simulink model "commpassbandmod"  (R2021b)
settings: Solver=VariableStepDiscrete  StartTime=0.0  StopTime=0.02  RelTol=1e-3  EnableMultiTasking=on
InitFcn:
  | commpassbandmodParams.Fc = 2.5e6;
  | commpassbandmodParams.F1 = commpassbandmodParams.Fc/3+.5e5;
undefined symbols (not defined in the file or in its folder): comm, constellation
libraries: commutil2 x3, dspsrcs4 x3, commdigbbndpm3 x2, commfilt2 x2, commchan3 x1, commsink2 x1, commrandsrc3 x1
Description:
  | Passband Modulation
  | 
  | This model shows a straightforward way to perform passband modulation, by multiplying a modulated complex signal with a complex sine wave to perform frequency upconversion.
settings Model: Creator=The MathWorks, Inc.  LastModifiedBy=The MathWorks, Inc.
settings SolverCC: AlgebraicLoopSolver=TrustRegion  InsertRTBMode=Auto
settings DataIOCC: LimitDataPoints=on  SaveFormat=Array  SaveOutput=off  SignalLogging=off  SaveTime=off  ReturnWorkspaceOutputs=off
settings OptimizationCC: ExpressionDepthLimit=2147483647  InitFltsAndDblsToZero=on  EfficientMapNaN2IntZero=off  LifeSpan=inf
settings DebuggingCC: UnderspecifiedInitializationDetection=Classic  MergeDetectMultiDrivingBlocksExec=none  SolverPrmCheckMsg=warning  FcnCallInpInsideContextMsg=warning  AllowSymbolicDim=off  StateNameClashWarn=warning  SFUnexpectedBacktrackingDiag=warning  SFNoUnconditionalDefaultTransitionDiag=warning  SFExecutionAtInitializationDiag=none  SFMachineParentedDataDiag=warning  ArithmeticOperatorsInVariantConditions=warning
settings HardwareCC: ProdBitPerPointer=32  ProdBitPerSizeT=32  ProdBitPerPtrDiffT=32  ProdLargestAtomicFloat=None  ProdIntDivRoundTo=Undefined  ProdEndianess=Unspecified  ProdWordSize=32  ProdHWDeviceType=32-bit Generic
settings ModelReferenceCC: PropagateSignalLabelsOutOfModel=off
settings SFSimCC: SimUseLocalCustomCode=off  CustomCodeUndefinedFunction=UseInterfaceOnly
settings RTWCC: RTWUseLocalCustomCode=off
settings CodeAppCC: StateflowObjectComments=on
settings GRTTargetCC: TargetLangStandard=C89/C90 (ANSI)  CombineOutputUpdateFcns=off  GRTInterface=on
settings ConfigComp: CovMetricSettings=dw  CovSaveCumulativeToWorkspaceVar=on  CovSaveSingleToWorkspaceVar=on  CovExternalEMLEnable=off  CovSFcnEnable=off

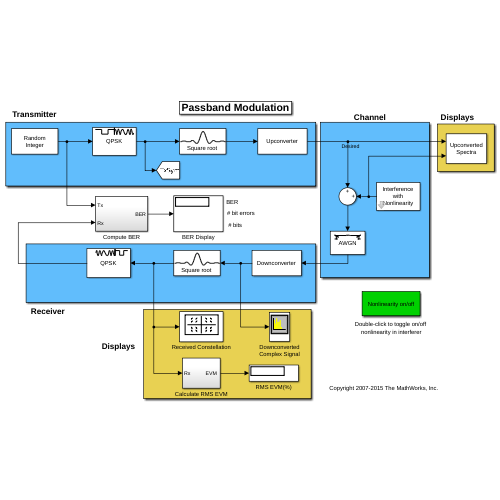
[thumbnail: Simulink's stored preview of the top-level diagram]
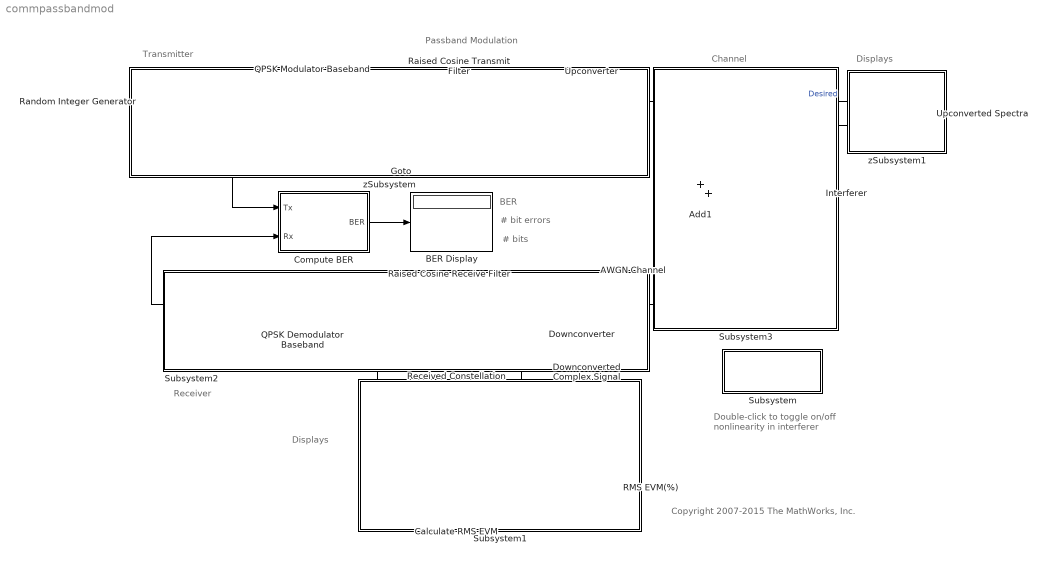
== system commpassbandmod ==
  note: Double-click to toggle on/off
      |  nonlinearity in interferer
  note: Passband Modulation
  note: Transmitter
  note: Receiver
  note: Channel
  note: Displays
  note: Displays
  note: BER
  note: # bit errors
  note: # bits
  note: Copyright 2007-2015 The MathWorks, Inc.
  AWGN Channel : commchan3/AWGN Channel  InputProcessing=Columns as channels (frame based)  seed=67  noiseMode="Signal to noise ratio  (Eb/No)"  EbNodB=8  EsNodB=10  SNRdB=10  bitsPerSym=2  Ps=1/(2*8)  Tsym=1e-6  variance=1
  Add1 : Sum  Inputs=|++
  BER Display : Display
  Calculate RMS EVM : Subsystem
  Compute BER : Subsystem
  Downconverted Complex Signal : SpectrumAnalyzer
  Downconverter : Subsystem
      mask Display: disp('Downconverter')
  Interferer : Subsystem  mask(Interference){nonlinOrder=3}
      mask prompts: nonlinOrder "Order of nonlinearity:"
      mask help: Generate out-of-band interference. Optionally process the interference with a third-order nonlinearity that creates an in-band harmonic.
      mask init:
      | if nonlinOrder == 1
      |     icontext = 'Interference\nwithout\nNonlinearity';
      | elseif nonlinOrder == 3
      |     icontext = 'Interference\nwith\nNonlinearity';
      | end
      mask Display: disp(icontext)
  QPSK Demodulator Baseband : commdigbbndpm3/QPSK Demodulator Baseband  OutType=Integer  DecType=Hard decision  VarSource=Dialog  Variance=1  Dec=Gray  Ph=pi/4  outDtype1=Inherit via internal rule  outDtype2=Inherit via internal rule  derotateFactorWordLen=16  derotateFactorDataTypeStr=Inherit: Same word length as input  derotateFactorLastDataTypeStr=Inherit: Same word length as input
  QPSK Modulator Baseband : commdigbbndpm3/QPSK Modulator Baseband  InType=Integer  Enc=Gray  Ph=pi/4  outDtype=double  outWordLen=16  outUDDataType=sfix(16)  outFracLenMode=Best precision  outFracLen=15  outDataTypeStr=double  outLastDataTypeStr=double
  RMS EVM(%) : Display
  Raised Cosine Receive Filter : commfilt2/Raised Cosine Receive Filter  filtType=Square root  R=0.2  filtSpan=8  N=8  downFactor=8  downOffset=0  filterGain=2  InputProcessing=Columns as channels (frame based)  RateOptions=Enforce single-rate processing  framing=Mute  checkCoeff=off  variableName=rcRxFilt1  currentFiltSpan=2*(4)  D=4  inputOffset=0  sampMode=Mute  saveAsFlag=0  rateMode=Downsampling  checkGain=User-specified  launchFVT=off  roundingMode=Floor  overflowMode=off  coeffDataTypeStr=Inherit: Same word length as input  coeffMin=[]  coeffMax=[]  coeffLastDataTypeStr=Inherit: Same word length as input  accumDataTypeStr=Inherit: Same as product output  accumLastDataTypeStr=Inherit: Same as product output  outputDataTypeStr=Inherit: Same as accumulator  outputMin=[]  outputMax=[]  outputLastDataTypeStr=Inherit: Same as accumulator
  Raised Cosine Transmit Filter : commfilt2/Raised Cosine Transmit Filter  filtType=Square root  R=0.2  filtSpan=8  N=8  filterGain=1  InputProcessing=Columns as channels (frame based)  RateOptions=Enforce single-rate processing  framing=Mute  checkCoeff=off  variableName=rcTxFilt1  checkGain=Normalized  sampMode=Mute  saveAsFlag=0  currentFiltSpan=2*(4)  D=4  launchFVT=off  roundingMode=Floor  overflowMode=off  coeffDataTypeStr=Inherit: Same word length as input  coeffMin=[]  coeffMax=[]  coeffLastDataTypeStr=Inherit: Same word length as input  outputDataTypeStr=Inherit: Same as accumulator  outputMin=[]  outputMax=[]  outputLastDataTypeStr=Inherit: Same as accumulator
  Random Integer Generator : commrandsrc3/Random Integer Generator  SetSize=4  SeedSource=Parameter  Seed=37  SampleTime=1e-6  SamplesPerFrame=100  OutputDataType=double  SimulateUsing=Interpreted execution
  Received Constellation : ConstellationDiagram  Tag=ScatterPlot
  Subsystem : Subsystem
      settings: OpenFcn=commpassbandmod_update
      mask Display: disp('Nonlinearity on/off')
  Subsystem1 : Subsystem
      mask Display: disp('')
  Subsystem2 : Subsystem
      mask Display: disp('')
  Subsystem3 : Subsystem
      mask Display: disp('')
  Upconverted Spectra : Subsystem
      mask Display: disp('Upconverted\nSpectra')
  Upconverter : Subsystem
      mask Display: disp('Upconverter')
  zSubsystem : Subsystem
      mask Display: disp('')
  zSubsystem1 : Subsystem
      mask Display: disp('')
  tag scope: TxSym=global
  wires:
  Random Integer Generator/1 -> QPSK Modulator Baseband/1, Compute BER/1(Tx)
  QPSK Modulator Baseband/1 -> Raised Cosine Transmit Filter/1, [TxSym]
  Compute BER/1(BER) -> BER Display/1
  QPSK Demodulator Baseband/1 -> Compute BER/2(Rx)
  AWGN Channel/1 -> Downconverter/1(In)
  Raised Cosine Transmit Filter/1 -> Upconverter/1(In)
  Raised Cosine Receive Filter/1 -> QPSK Demodulator Baseband/1, Calculate RMS EVM/1(Rx), Received Constellation/1
  Downconverter/1(Out) -> Raised Cosine Receive Filter/1, Downconverted Complex Signal/1
  Add1/1 -> AWGN Channel/1
  Calculate RMS EVM/1("EVM ") -> RMS EVM(%)/1
  Upconverter/1(Out) -> Add1/1, Upconverted Spectra/1(In1)  "Desired"
  Interferer/1(Out1) -> Add1/2, Upconverted Spectra/2(In2)

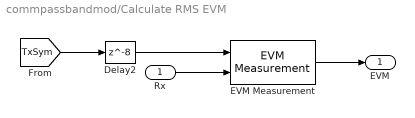
== system commpassbandmod/Calculate RMS EVM ==
  Rx : Inport
  Delay2 : Delay  DelayLength=8  InitialCondition=1  InputProcessing=Columns as channels (frame based)
  EVM Measurement : commutil2/EVM Measurement  Normalization=Average reference signal power  AverageConstellationPower=1  PeakConstellationPower=1  ReferenceSignalSource=Input port  ReferenceConstellation=constellation( comm.QPSKModulator )  MeasurementIntervalSource=Input length  MeasurementInterval=100  AveragingDimensions=1  MaximumEVMOutputPort=off  XPercentileEVMOutputPort=off  XPercentileValue=95  SymbolCountOutputPort=off  SimulateUsing=Interpreted execution
      settings: SourceProductBaseCode=CM
  "EVM " : Outport  VectorParamsAs1DForOutWhenUnconnected=off
  wires:
  Delay2/1 -> EVM Measurement/1
  [TxSym] -> Delay2/1
  Rx/1 -> EVM Measurement/2
  EVM Measurement/1 -> "EVM "/1

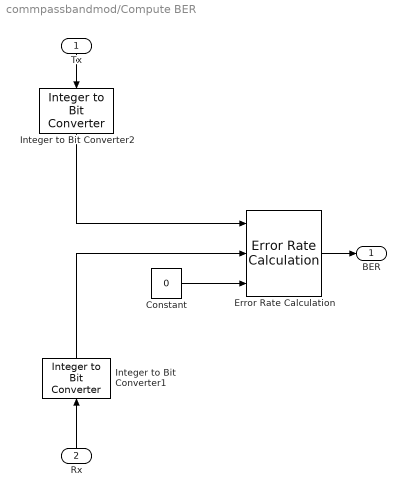
== system commpassbandmod/Compute BER ==
  Tx : Inport
  Rx : Inport  Port=2
  Constant : Constant  Value=0  SampleTime=1e-4
  Error Rate Calculation : commsink2/Error Rate Calculation  N=16  st_delay=0  cp_mode=Entire frame  subframe=[]  PMode=Port  WsName=ErrorVec  RsMode2=on  stop=off  numErr=100  maxBits=1e6
  Integer to Bit Converter1 : commutil2/Integer to Bit Converter  nbits=2  signedInputValues=Unsigned  bitOrder=MSB first  outDtype=boolean
  Integer to Bit Converter2 : commutil2/Integer to Bit Converter  nbits=2  signedInputValues=Unsigned  bitOrder=MSB first  outDtype=boolean
  BER : Outport  VectorParamsAs1DForOutWhenUnconnected=off
  wires:
  Integer to Bit Converter2/1 -> Error Rate Calculation/1
  Integer to Bit Converter1/1 -> Error Rate Calculation/2
  Tx/1 -> Integer to Bit Converter2/1
  Error Rate Calculation/1 -> BER/1
  Rx/1 -> Integer to Bit Converter1/1
  Constant/1 -> Error Rate Calculation/3

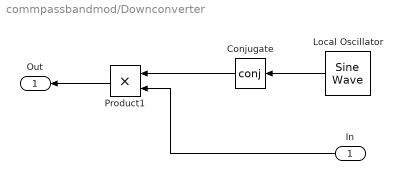
== system commpassbandmod/Downconverter ==
  In : Inport
  Conjugate : Math  Operator=conj  SignedPower=on  SaturateOnIntegerOverflow=on
  Local Oscillator : dspsrcs4/Sine Wave  Amplitude=1  Frequency=commpassbandmodParams.Fc  Phase=0  SampleMode=Discrete  OutComplex=Complex  CompMethod=Trigonometric fcn  TableSize=Speed  SampleTime=(1e-6) /8  SamplesPerFrame=800  ResetState=Restart at time zero  OutputFrames=off  dataType=double  wordLen=16  udDataType=sfix(16)  fracBitsMode=Best precision  numFracBits=15  OutDataTypeStr=double  LastOutDataTypeStr=double
  Product1 : Product  RndMeth=Zero
  Out : Outport  VectorParamsAs1DForOutWhenUnconnected=off
  wires:
  Conjugate/1 -> Product1/1
  Product1/1 -> Out/1
  In/1 -> Product1/2
  Local Oscillator/1 -> Conjugate/1

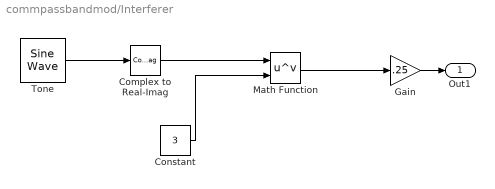
== system commpassbandmod/Interferer ==
  Complex to Real-Imag : ComplexToRealImag  Output=Real
  Constant : Constant  Value=3
  Gain : Gain  Gain=.25
  Math Function : Math  Operator=pow  SignedPower=on  SaturateOnIntegerOverflow=on
  "Tone " : dspsrcs4/Sine Wave  Amplitude=1  Frequency=commpassbandmodParams.F1  Phase=0  SampleMode=Discrete  OutComplex=Complex  CompMethod=Trigonometric fcn  TableSize=Speed  SampleTime=(1e-6) /8  SamplesPerFrame=800  ResetState=Restart at time zero  OutputFrames=off  dataType=double  wordLen=16  udDataType=sfix(16)  fracBitsMode=Best precision  numFracBits=15  OutDataTypeStr=double  LastOutDataTypeStr=double
  Out1 : Outport  VectorParamsAs1DForOutWhenUnconnected=off
  wires:
  Complex to Real-Imag/1 -> Math Function/1
  Constant/1 -> Math Function/2
  "Tone "/1 -> Complex to Real-Imag/1
  Math Function/1 -> Gain/1
  Gain/1 -> Out1/1

== system commpassbandmod/Subsystem ==

== system commpassbandmod/Subsystem1 ==

== system commpassbandmod/Subsystem2 ==

== system commpassbandmod/Subsystem3 ==

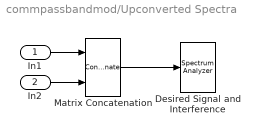
== system commpassbandmod/Upconverted Spectra ==
  In1 : Inport
  In2 : Inport  Port=2
  Desired Signal and Interference : SpectrumAnalyzer
  Matrix Concatenation : Concatenate  Mode=Multidimensional array  ConcatenateDimension=2
  wires:
  Matrix Concatenation/1 -> Desired Signal and Interference/1
  In1/1 -> Matrix Concatenation/1
  In2/1 -> Matrix Concatenation/2

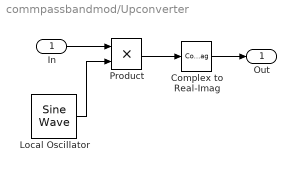
== system commpassbandmod/Upconverter ==
  In : Inport
  Complex to Real-Imag : ComplexToRealImag  Output=Real
  Local Oscillator : dspsrcs4/Sine Wave  Amplitude=1  Frequency=commpassbandmodParams.Fc  Phase=0  SampleMode=Discrete  OutComplex=Complex  CompMethod=Trigonometric fcn  TableSize=Speed  SampleTime=(1e-6) /8  SamplesPerFrame=800  ResetState=Restart at time zero  OutputFrames=off  dataType=double  wordLen=16  udDataType=sfix(16)  fracBitsMode=Best precision  numFracBits=15  OutDataTypeStr=double  LastOutDataTypeStr=double
  Product : Product  RndMeth=Zero
  Out : Outport  VectorParamsAs1DForOutWhenUnconnected=off
  wires:
  Complex to Real-Imag/1 -> Out/1
  Product/1 -> Complex to Real-Imag/1
  Local Oscillator/1 -> Product/2
  In/1 -> Product/1

== system commpassbandmod/zSubsystem ==

== system commpassbandmod/zSubsystem1 ==
